simulink model "obstacleAvoidance_uTurn_solution"  (R2017a)
settings: Solver=FixedStepDiscrete  StartTime=0.0  StopTime=10  FixedStep=0.01  RelTol=1e-3
InitFcn:
  | Ts = 0.01;
  | axleLength = 0.28;
  | wheelR = 0.052;
  | load wheelMotorModel
  | load wheelMotorLUT
undefined symbols (not defined in the file): motorIp, motorSp, ticksPerDeg, ticksPerRot
libraries: mobileRoboticsTrainingLib x6, simulink_extras x1
settings Model: Creator=sseshadr  LastModifiedBy=shiremat

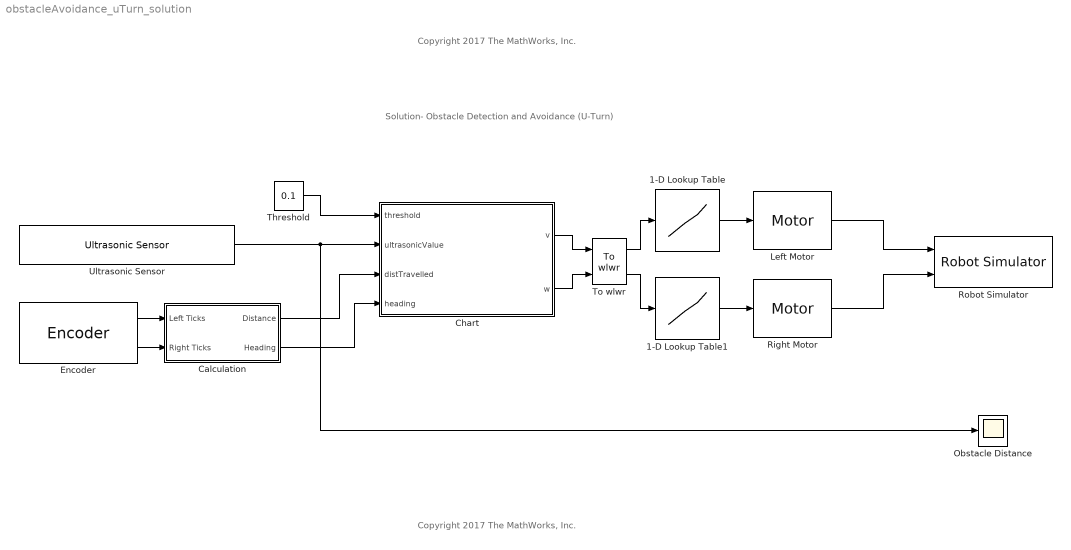
== system obstacleAvoidance_uTurn_solution ==
  note: Solution- Obstacle Detection and Avoidance (U-Turn)
  note: Copyright 2017 The MathWorks, Inc.
  note: Copyright 2017 The MathWorks, Inc.
  1-D Lookup Table : Lookup_n-D  NumberOfTableDimensions=1  BreakpointsForDimension1=motorSp  Table=motorIp  ExtrapMethod=Clip  InternalRulePriority=Speed  RndMeth=Simplest  InputSameDT=on
  1-D Lookup Table1 : Lookup_n-D  NumberOfTableDimensions=1  BreakpointsForDimension1=motorSp  Table=motorIp  ExtrapMethod=Clip  InternalRulePriority=Speed  RndMeth=Simplest  InputSameDT=on
  Calculation : Subsystem
  Chart : Stateflow chart  TreatAsAtomicUnit=on
  Encoder : mobileRoboticsTrainingLib/Encoder  axleLength=axleLength  wheelR=wheelR  ticksPerRot=ticksPerRot
      settings: SourceProductName=Mobile Robotics Training Library
  Left Motor : mobileRoboticsTrainingLib/Motor  motorPlant=wheelMotorModel  sensorType=Speed
      settings: SourceProductName=Mobile Robotics Training Library
  Obstacle Distance : Scope
  Right Motor : mobileRoboticsTrainingLib/Motor  motorPlant=wheelMotorModel  sensorType=Speed
      settings: SourceProductName=Mobile Robotics Training Library
  Robot Simulator : mobileRoboticsTrainingLib/Robot Simulator  Priority=99  mapVar=mapForSim  startX=2.5675  startY=.9  startTheta=90  axleLength=axleLength  wheelR=wheelR
  Threshold : Constant  Value=0.1
  To wlwr : mobileRoboticsTrainingLib/To wlwr  axleLength=axleLength  wheelR=wheelR
  Ultrasonic Sensor : mobileRoboticsTrainingLib/Ultrasonic Sensor  mapVar=mapForSim  maxSenRange=2  minSenRange=0.02  senRes=0.02  sensOff=[0 0]
      settings: SourceProductName=Mobile Robotics Training Library
  wires:
  Left Motor/1 -> Robot Simulator/1
  1-D Lookup Table1/1 -> Right Motor/1
  1-D Lookup Table/1 -> Left Motor/1
  Right Motor/1 -> Robot Simulator/2
  To wlwr/1 -> 1-D Lookup Table/1
  To wlwr/2 -> 1-D Lookup Table1/1
  Chart/1(v) -> To wlwr/1
  Ultrasonic Sensor/1 -> Obstacle Distance/1, Chart/2(ultrasonicValue)
  Threshold/1 -> Chart/1(threshold)
  Chart/2(w) -> To wlwr/2
  Calculation/1(Distance) -> Chart/3(distTravelled)
  Encoder/2 -> Calculation/2(Right Ticks)
  Encoder/1 -> Calculation/1(Left Ticks)
  Calculation/2(Heading) -> Chart/4(heading)

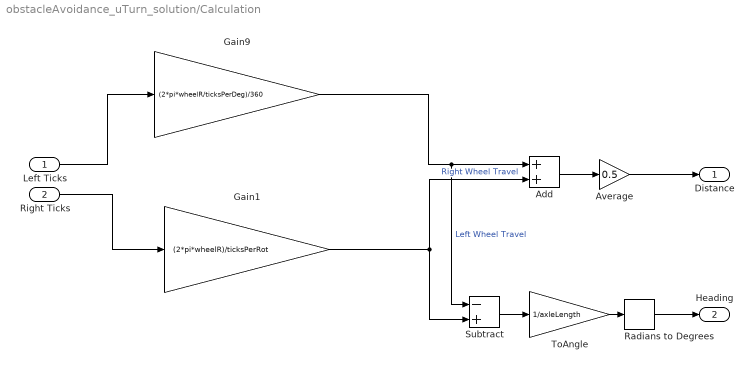
== system obstacleAvoidance_uTurn_solution/Calculation ==
  Left Ticks : Inport
  Right Ticks : Inport  Port=2
  Add : Sum
  Average : Gain  Gain=0.5
  Gain1 : Gain  Gain=(2*pi*wheelR)/ticksPerRot
  Gain9 : Gain  Gain=(2*pi*wheelR/ticksPerDeg)/360
  Radians to Degrees : simulink_extras/Transformations/Radians to Degrees
  Subtract : Sum  Inputs=-+
  ToAngle : Gain  Gain=1/axleLength
  Distance : Outport
  Heading : Outport  Port=2
  wires:
  Average/1 -> Distance/1
  Add/1 -> Average/1
  Gain9/1 -> Add/1, Subtract/1  "Left Wheel Travel"
  Right Ticks/1 -> Gain1/1
  Left Ticks/1 -> Gain9/1
  Gain1/1 -> Subtract/2, Add/2  "Right Wheel Travel"
  Subtract/1 -> ToAngle/1
  ToAngle/1 -> Radians to Degrees/1
  Radians to Degrees/1 -> Heading/1

== stateflow chart obstacleAvoidance_uTurn_solution/Chart ==
  state Go
    entry:
    v = 0.2;
    w=0;
  state Pause
    entry: v = 0;
  note: %Turn 180 degrees
  state Reverse
    entry:
    v = -0.2;
    distNow = distTravelled;
  state U_Turn
    entry:
    v = 0; w = 1.5;
    headingNow= heading;
  note: %Reverse for 5 cms
  (default) -> Go
  Go -> Pause : [ultrasonicValue <= threshold && ultrasonicValue > 0]
  Pause -> Go [order 1] : [ultrasonicValue > threshold]
  U_Turn -> Go : [heading > headingNow +180]
  Pause -> Reverse [order 2] : after(2,sec)
  Reverse -> U_Turn : [distTravelled < distNow - 0.05]
  data: threshold input; ultrasonicValue input; distTravelled input; v output; heading input; w output; distNow local; headingNow local
